simulink model "DC_equivalent_simulation"  (R2021a)
settings: Solver=VariableStepAuto  StartTime=0.0  StopTime=0.001  RelTol=1e-3
values from neighbouring files (symbols this model uses):
  R = 50    [DC_equivalent_circuit.m]
  R_g = 50*10^6    (= 50000000)    [DC_equivalent_circuit.m]
  R_sh = 50    [DC_equivalent_circuit.m]
libraries: fl_lib x25, nesl_utility x8
settings Model: Creator=jsm_9  LastModifiedBy=jsm_9

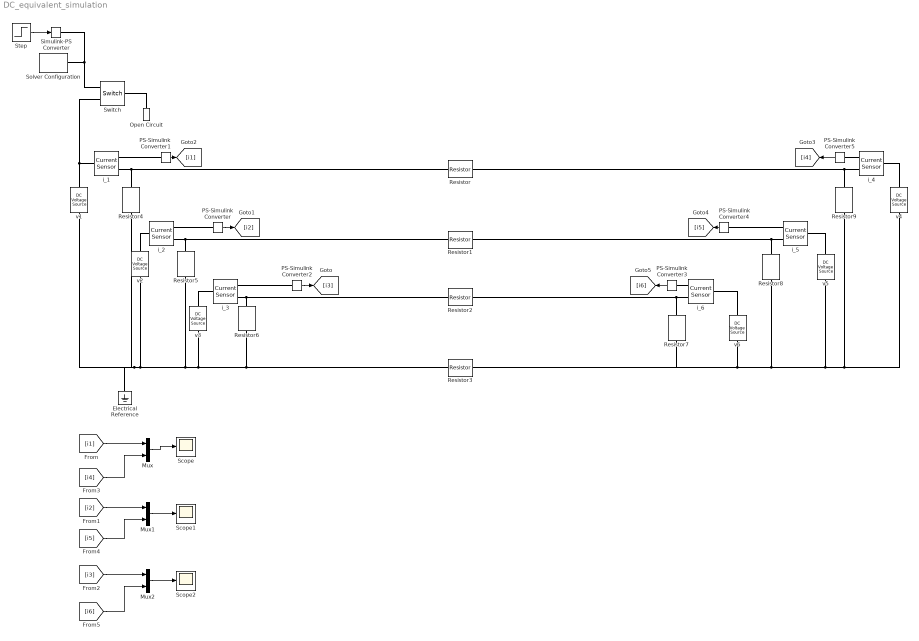
== system DC_equivalent_simulation ==
  Electrical Reference : fl_lib/Electrical/Electrical Elements/Electrical Reference
  Mux : Mux  Inputs=2
  Mux1 : Mux  Inputs=2
  Mux2 : Mux  Inputs=2
  Open Circuit : fl_lib/Electrical/Electrical Elements/Open Circuit  v_specify=off  v_priority=None  v=0 V  v_nominal_specify=off  v_nominal_unit=V  v_nominal_value=1
      settings: SourceProductBaseCode=SS
  PS-Simulink Converter{,1..5} (6 alike) : nesl_utility/PS-Simulink Converter  PhysicalDomain=network_engine_domain  SubClassName=ps_output  LeftPortType=input  RightPortType=output  PseudoPeriodic=off  Frequencies=[]  Unit=inherit  AffineConversion=off
      settings: SourceProductBaseCode=PW,SS
  Resistor : fl_lib/Electrical/Electrical Elements/Resistor  R=R Ohm  i_specify=off  i_priority=None  i=0 A  i_nominal_specify=off  i_nominal_unit=A  i_nominal_value=1  v_specify=off  v_priority=None  v=0 V  v_nominal_specify=off  v_nominal_unit=V  v_nominal_value=1
  Resistor1 : fl_lib/Electrical/Electrical Elements/Resistor  R=R Ohm  i_specify=off  i_priority=None  i=0 A  i_nominal_specify=off  i_nominal_unit=A  i_nominal_value=1  v_specify=off  v_priority=None  v=0 V  v_nominal_specify=off  v_nominal_unit=V  v_nominal_value=1
  Resistor2 : fl_lib/Electrical/Electrical Elements/Resistor  R=R Ohm  i_specify=off  i_priority=None  i=0 A  i_nominal_specify=off  i_nominal_unit=A  i_nominal_value=1  v_specify=off  v_priority=None  v=0 V  v_nominal_specify=off  v_nominal_unit=V  v_nominal_value=1
  Resistor3 : fl_lib/Electrical/Electrical Elements/Resistor  R=R_sh Ohm  i_specify=off  i_priority=None  i=0 A  i_nominal_specify=off  i_nominal_unit=A  i_nominal_value=1  v_specify=off  v_priority=None  v=0 V  v_nominal_specify=off  v_nominal_unit=V  v_nominal_value=1
  Resistor{4..9} (6 alike) : fl_lib/Electrical/Electrical Elements/Resistor  R=R_g Ohm  i_specify=off  i_priority=None  i=0 A  i_nominal_specify=off  i_nominal_unit=A  i_nominal_value=1  v_specify=off  v_priority=None  v=0 V  v_nominal_specify=off  v_nominal_unit=V  v_nominal_value=1
  Scope : Scope
  Scope1 : Scope
  Scope2 : Scope
  Simulink-PS Converter : nesl_utility/Simulink-PS Converter  PhysicalDomain=network_engine_domain  SubClassName=ps_input  LeftPortType=input  RightPortType=output  PseudoPeriodic=off  Frequencies=[]  NoiseDistribution=none  NoiseParameters=[]  Unit=1  AffineConversion=off  FilteringAndDerivatives=provide  SimscapeFilterOrder=1  InputFilterTimeConstant=0.001  UdotUserProvided=0
      settings: SourceProductBaseCode=PW,SS
  Solver Configuration : nesl_utility/Solver Configuration  PhysicalDomain=network_engine_domain  SubClassName=solver  LeftPortType=input  RightPortType=generic  Tones=[]  Harmonics=[]  SimulateNoise=off  Profile=off  UseLocalSampling=off  EnableSwitchedLinearOptims=on  FrequencyDomain=off  UseCCode=off  RelTol=0.001  AbsTol=1e-06  MinStep=1e-09  ToWorkspace=off  RevertToSquareIcSolve=off  NumHomotopyIterations=100  PhasorMode=off  PhasorModeNumHarmonics=1  DoDC=off  ResidualTolerance=1e-09  UseLocalSolver=off  LocalSolverChoice=NE_BACKWARD_EULER_ADVANCER  LocalSolverSampleTime=0.001  DoFixedCost=off  MaxNonlinIter=3  MaxModeIter=2  ComputeImpulses=off  ImpulseIterations=2  LinearAlgebra=auto  EquationFormulation=NE_TIME_EF  DelaysMemoryBudget=1024  AutomaticFiltering=on  FilteringTimeConstant=0.001  PartitionStorageMethod=AS_NEEDED  PartitionMemoryBudget=1024  PartitionMethod=ROBUST
      settings: SourceProductBaseCode=PW,SS
  Step : Step  SampleTime=0
  Switch : fl_lib/Electrical/Electrical Elements/Switch  R_closed=0.01 Ohm  G_open=1e-8 1/Ohm  Threshold=0.5  i_specify=off  i_priority=None  i=0 A  i_nominal_specify=off  i_nominal_unit=A  i_nominal_value=1  v_specify=off  v_priority=None  v=0 V  v_nominal_specify=off  v_nominal_unit=V  v_nominal_value=1
  i_{1..6} (6 alike) : fl_lib/Electrical/Electrical Sensors/Current Sensor
  v1 : fl_lib/Electrical/Electrical Sources/DC Voltage Source  v0=V1 V
  v2 : fl_lib/Electrical/Electrical Sources/DC Voltage Source  v0=V2 V
  v3 : fl_lib/Electrical/Electrical Sources/DC Voltage Source  v0=V3 V
  v4 : fl_lib/Electrical/Electrical Sources/DC Voltage Source  v0=V4 V
  v5 : fl_lib/Electrical/Electrical Sources/DC Voltage Source  v0=V5 V
  v6 : fl_lib/Electrical/Electrical Sources/DC Voltage Source  v0=V6 V
  wires:
  Step/1 -> Simulink-PS Converter/1
  PS-Simulink Converter1/1 -> [i1]
  PS-Simulink Converter/1 -> [i2]
  PS-Simulink Converter5/1 -> [i4]
  PS-Simulink Converter4/1 -> [i5]
  [i1] -> Mux/1
  PS-Simulink Converter3/1 -> [i6]
  Mux/1 -> Scope/1
  Mux2/1 -> Scope2/1
  Mux1/1 -> Scope1/1
  [i4] -> Mux/2
  [i2] -> Mux1/1
  [i5] -> Mux1/2
  [i3] -> Mux2/1
  [i6] -> Mux2/2
  PS-Simulink Converter2/1 -> [i3]
  connections:
  Resistor6/RConn1 -- v1/RConn1 -- Electrical Reference/LConn1 -- Resistor4/RConn1 -- v2/RConn1 -- Resistor5/RConn1 -- v3/RConn1 -- Resistor3/LConn1
  i_3/RConn2 -- Resistor6/LConn1 -- Resistor2/LConn1
  v3/LConn1 -- i_3/LConn1
  Resistor1/LConn1 -- Resistor5/LConn1 -- i_2/RConn2
  i_2/LConn1 -- v2/LConn1
  i_1/LConn1 -- Switch/RConn2 -- v1/LConn1
  i_1/RConn2 -- Resistor4/LConn1 -- Resistor/LConn1
  Resistor9/RConn1 -- v5/RConn1 -- v6/RConn1 -- Resistor7/RConn1 -- Resistor3/RConn1 -- Resistor8/RConn1 -- v4/RConn1
  i_6/RConn2 -- Resistor7/LConn1 -- Resistor2/RConn1
  i_5/RConn2 -- Resistor8/LConn1 -- Resistor1/RConn1
  i_4/RConn2 -- Resistor/RConn1 -- Resistor9/LConn1
  Switch/LConn1 -- Open Circuit/LConn1
  Simulink-PS Converter/RConn1 -- Solver Configuration/RConn1 -- Switch/RConn1
  i_1/RConn1 -- PS-Simulink Converter1/LConn1
  PS-Simulink Converter/LConn1 -- i_2/RConn1
  PS-Simulink Converter5/LConn1 -- i_4/RConn1
  PS-Simulink Converter4/LConn1 -- i_5/RConn1
  i_3/RConn1 -- PS-Simulink Converter2/LConn1
  PS-Simulink Converter3/LConn1 -- i_6/RConn1
  i_6/LConn1 -- v6/LConn1
  i_5/LConn1 -- v5/LConn1
  i_4/LConn1 -- v4/LConn1
